simulink subsystem "pseudoInverseMatrix"  (R2024b)
settings: Solver=VariableStepAuto  StartTime=0.0  StopTime=10.0  RelTol=1e-3
settings Model: Creator=ricca  LastModifiedBy=ricca

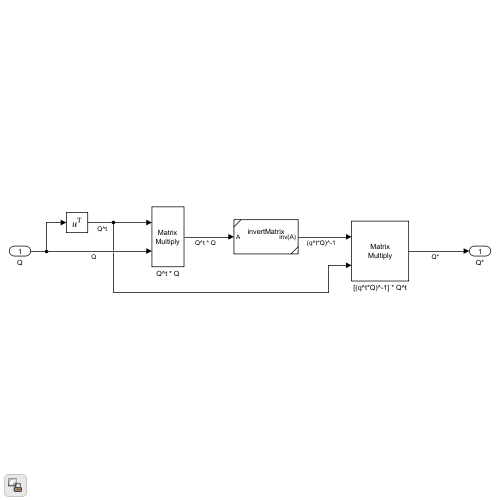
[thumbnail: Simulink's stored preview of the top-level diagram]
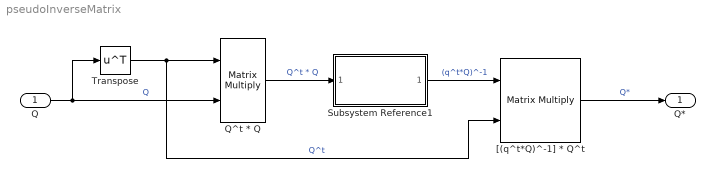
== system pseudoInverseMatrix ==
  Q : Inport
  Q^t * Q : Product  Multiplication=Matrix(*)
  Subsystem Reference1 : Subsystem  ReferencedSubsystem=invertMatrix
  Transpose : Math  Operator=transpose
  "[(q^t*Q)^-1] * Q^t" : Product  Multiplication=Matrix(*)
  Q* : Outport
  wires:
  Q/1 -> Transpose/1, Q^t * Q/2  "Q"
  Transpose/1 -> Q^t * Q/1, "[(q^t*Q)^-1] * Q^t"/2  "Q^t"
  Q^t * Q/1 -> Subsystem Reference1/1  "Q^t * Q"
  Subsystem Reference1/1 -> "[(q^t*Q)^-1] * Q^t"/1  "(q^t*Q)^-1"
  "[(q^t*Q)^-1] * Q^t"/1 -> Q*/1  "Q*"
